simulink subsystem "Batery_Bhv"  (R2024b)
settings: Solver=VariableStepAuto  StartTime=0.0  StopTime=10.0  RelTol=1e-3
libraries: simulink x2
settings Model: Creator=m4ttn  LastModifiedBy=m4ttn

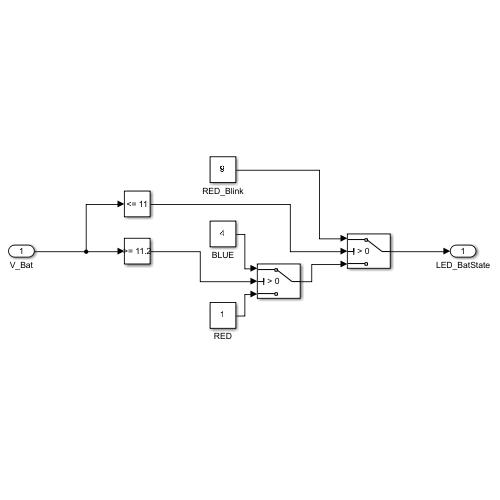
[thumbnail: Simulink's stored preview of the top-level diagram]
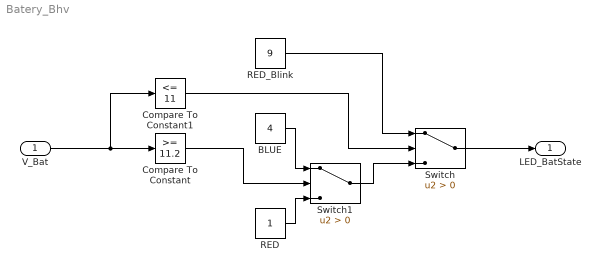
== system Batery_Bhv ==
  V_Bat : Inport
  BLUE : Constant  Value=4  OutDataTypeStr=uint8
  Compare To Constant : simulink/Logic and Bit Operations/Compare To Constant  relop=>=  const=11.2  OutDataTypeStr=boolean
  Compare To Constant1 : simulink/Logic and Bit Operations/Compare To Constant  relop=<=  const=11  OutDataTypeStr=boolean
  RED : Constant  OutDataTypeStr=uint8
  RED_Blink : Constant  Value=9  OutDataTypeStr=uint8
  Switch : Switch  Criteria=u2 > Threshold  OutDataTypeStr=uint8  SaturateOnIntegerOverflow=off  InputSameDT=off
  Switch1 : Switch  Criteria=u2 > Threshold  SaturateOnIntegerOverflow=off  InputSameDT=off
  LED_BatState : Outport  OutDataTypeStr=uint8
  wires:
  V_Bat/1 -> Compare To Constant/1, Compare To Constant1/1
  Switch1/1 -> Switch/3
  Compare To Constant/1 -> Switch1/2
  RED/1 -> Switch1/3
  BLUE/1 -> Switch1/1
  RED_Blink/1 -> Switch/1
  Switch/1 -> LED_BatState/1
  Compare To Constant1/1 -> Switch/2
